simulink model "CurrDrvSensCombo_Test"  (R2025b)
settings: Solver=FixedStepDiscrete  StartTime=0.0  StopTime=Inf  FixedStep=0.01  RelTol=1e-3
undefined symbols (not defined in the file): X, Y
libraries: MagLevTbx_BaseLib x8, simulink x1
settings Model: SimulationMode=external  ExtModeTrigDuration=2  Creator=riccardo  LastModifiedBy=riccardo
settings SolverCC: AutoInsertRateTranBlk=on
settings OptimizationCC: EnhancedBackFolding=on  PassReuseOutputArgsAs=Individual arguments  ZeroExternalMemoryAtStartup=off  ZeroInternalMemoryAtStartup=off  MaxStackSize=64  OptimizeBlockOrder=speed  DifferentSizesBufferReuse=on  OptimizationCustomize=off  EfficientTunableParamExpr=on
settings DebuggingCC: ParameterTunabilityLossMsg=error
settings HardwareCC: ProdBitPerPointer=32.0  ProdBitPerSizeT=32.0  ProdBitPerPtrDiffT=32.0  ProdLargestAtomicInteger=Long  ProdLargestAtomicFloat=Double  ProdWordSize=32.0  ProdHWDeviceType=ARM Compatible->ARM Cortex
settings SFSimCC: MATLABDynamicMemAlloc=off
settings RTWCC: SystemTargetFile=ert.tlc  HardwareBoard=Teensy 4.1 (Arduino Compatible)  TemplateMakefile=ert_default_tmf  Toolchain=Arduino ARM M7  BuildConfiguration=Faster Runs  Description=Embedded Coder
settings CodeAppCC: ForceParamTrailComments=on  IgnoreCustomStorageClasses=off  OperatorAnnotations=on  SimulinkDataObjDesc=on  SFDataObjDesc=on  InsertBlockDesc=on
settings ERTTargetCC: ExtModeTransport=3.0  ExtModeStaticAlloc=on  ExtModeAutomaticAllocSize=off  ExtModeStaticAllocSize=65536.0  ExtModeMexFile=ext_xcp  ExtModeIntrfLevel=Level2 - Open  InlinedParameterPlacement=Hierarchical  RootIOFormat=Structure reference  TargetLangStandard=C99 (ISO)  SupportContinuousTime=on  SupportVariableSizeSignals=on

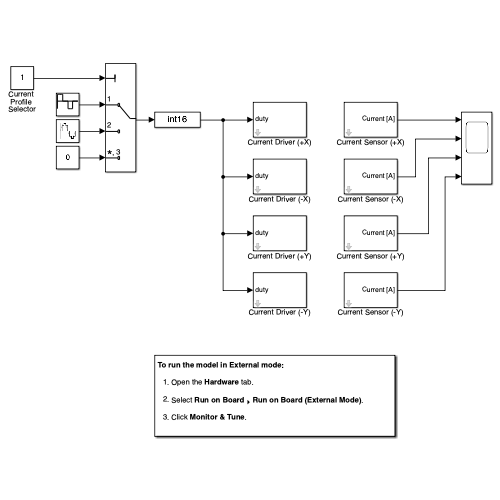
[thumbnail: Simulink's stored preview of the top-level diagram]
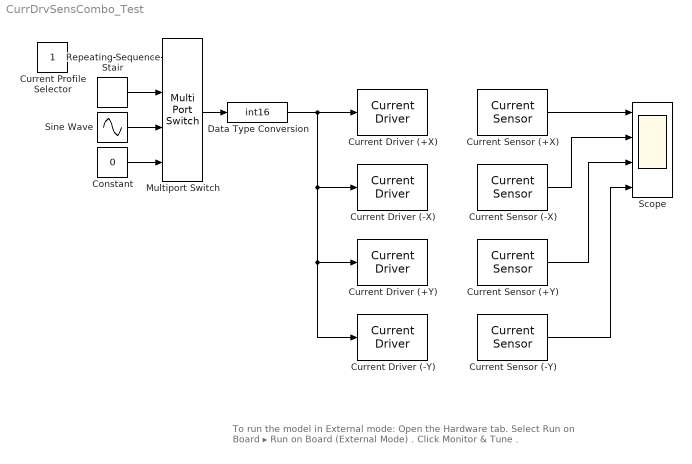
== system CurrDrvSensCombo_Test ==
  note: To run the model in External mode:
      | Open the Hardware tab.
      | Select Run on Board ▸ Run on Board (External Mode) .
      | Click Monitor & Tune .
  Constant : Constant  Value=0
  Current Profile Selector : Constant
  Current Driver (+X) : MagLevTbx_BaseLib/Outputs/Current Driver  driverId=+X  sampleTime=-1  showEnablePort=off
      settings: SourceProductName=MagLev Toolbox
  Current Driver (+Y) : MagLevTbx_BaseLib/Outputs/Current Driver  driverId=+Y  sampleTime=-1  showEnablePort=off
      settings: SourceProductName=MagLev Toolbox
  Current Driver (-X) : MagLevTbx_BaseLib/Outputs/Current Driver  driverId=-X  sampleTime=-1  showEnablePort=off
      settings: SourceProductName=MagLev Toolbox
  Current Driver (-Y) : MagLevTbx_BaseLib/Outputs/Current Driver  driverId=-Y  sampleTime=-1  showEnablePort=off
      settings: SourceProductName=MagLev Toolbox
  Current Sensor (+X) : MagLevTbx_BaseLib/Inputs/Current Sensor  sensorId=+X  sampleTime=-1  showEnablePort=off
      settings: SourceProductName=MagLev Toolbox
  Current Sensor (+Y) : MagLevTbx_BaseLib/Inputs/Current Sensor  sensorId=+Y  sampleTime=-1  showEnablePort=off
      settings: SourceProductName=MagLev Toolbox
  Current Sensor (-X) : MagLevTbx_BaseLib/Inputs/Current Sensor  sensorId=-X  sampleTime=-1  showEnablePort=off
      settings: SourceProductName=MagLev Toolbox
  Current Sensor (-Y) : MagLevTbx_BaseLib/Inputs/Current Sensor  sensorId=-Y  sampleTime=-1  showEnablePort=off
      settings: SourceProductName=MagLev Toolbox
  Data Type Conversion : DataTypeConversion  OutDataTypeStr=int16  SaturateOnIntegerOverflow=off  RndMeth=Floor
  Multiport Switch : MultiPortSwitch  SaturateOnIntegerOverflow=off  InputSameDT=off
  Repeating Sequence Stair : simulink/Sources/Repeating Sequence Stair  OutValues=[32 32 32 32 0 0 0 0 -32 -32 -32 -32 0 0 0 0].'  tsamp=0.1  OutMin=[]  OutMax=[]  OutDataTypeStr=double  OutputDataTypeScalingMode=double  OutDataType=fixdt(0,8)  ConRadixGroup=Best Precision: Vector-wise  OutScaling=2^-12
  Scope : Scope  NumInputPorts=4
      settings: ActiveDisplayYMinimum=-0.0016129176510730758  ActiveDisplayYMaximum=0.0037634214531863108
  Sine Wave : Sin  Amplitude=32  Frequency=2*pi*0.25  SampleTime=0.01
  wires:
  Repeating Sequence Stair/1 -> Multiport Switch/2
  Sine Wave/1 -> Multiport Switch/3
  Constant/1 -> Multiport Switch/4
  Current Profile Selector/1 -> Multiport Switch/1
  Multiport Switch/1 -> Data Type Conversion/1
  Current Sensor (+X)/1 -> Scope/1
  Current Sensor (-X)/1 -> Scope/2
  Current Sensor (+Y)/1 -> Scope/3
  Current Sensor (-Y)/1 -> Scope/4
  Data Type Conversion/1 -> Current Driver (+X)/1, Current Driver (+Y)/1, Current Driver (-Y)/1, Current Driver (-X)/1
